simulink model "Intergration_ACC"  (R2018b)
settings: Solver=FixedStepDiscrete  StartTime=0.0  StopTime=inf  FixedStep=0.005  RelTol=1e-3
PostLoadFcn:
  | if any(exist('dsrtsu_mdlpostloadfcn', 'file') ~= 0), dsrtsu_mdlpostloadfcn('Execute', bdroot); end
values from neighbouring files (symbols this model uses):
  P_x165_On = 1.0    [CAN_Tx.sldd]
  P_x242_On = 1.0    [CAN_Tx.sldd]
  P_x246_On = 1.0    [CAN_Tx.sldd]
libraries: rtican x112, simulink x59
(part 25 of 31)

== system Intergration_ACC/TX/ESC_FrontWheelSpeedKPH_0x123 ==
  <WhlGndVelLDrvn_Radar> : Inport
  <WhlGndVelRDrvn_Radar> : Inport  Port=2
  <LDrvnWhlRotlDircn> : Inport  Port=3
  <RDrvnWhlRotlDircn> : Inport  Port=4
  Cast To Double{1..6} (6 alike) : DataTypeConversion  OutDataTypeStr=double
  Constant : Constant  Value=0  OutDataTypeStr=uint8
  Constant1 : Constant  Value=0  OutDataTypeStr=double
  Constant6 : Constant  Value=7  OutDataTypeStr=uint8
  ESC_FrontWheelSpeedKPH : rtican/RTICAN Transmit (TX)   Reserved1=[]  Reserved2=[]  Reserved3=[]  Reserved4=[]  SfcnMessage=[]  Msg_Struct=[]  BoardTypeNo=[]  BoardNo=[]  ChannelNo=[]  Parameters=[]  DialogFcn=[]  UnitName=[]  Revision=[]  UnitValues=[]  DSProperties=struct('RTI',struct('Version',uint32(5),'BlockType',struct('isSLSource',uint8(1),'isSLSink',uint8(1),'isHWSource',uint8(0),'isHWSink',uint8(0),'isSetup',uint8(0),'isInline',uint8(1),'isNonInline',uint8(0),'isInterrupt',uint8(0),'isChannelwise',uint8(0)),'IOBoardType','RTICAN','UnitType','MESSAGE','Identifier','TX','DialogType','MSVC','BlockSet','RTICAN','SlaveProcessor','CAN'))  RTIBlockInterface=struct('InputPortsWidth',int32([1 1 1 1 1 1 1 1 1 1]),'InputPortsActive',[1 1 1 1 1 1 1 1 1 1],'InputPortsName',{{'ESC_FrontWheelSpeedsKPH_Checksum','ESC_FrontWheelSpeedsKPH_AliveCou','ESC_Mcylinder_PressureInvalid','ESC_Mcylinder_Pressure','ESC_FRWheelSpeedInvalid','ESC_FRWheelDirection','ESC_FRWheelSpeedKPH','ESC_FLWheelSpeedInvalid','ESC_FLWheelDirection','ESC_FLWheelSpeedKPH'}},'InputPortsDataType',{{'SS_DOUBLE','SS_DOUBLE','SS_DOUBLE','SS_DOUBLE','SS_DOUBLE','SS_DOUBLE','SS_DOUBLE','SS_DOUBLE','SS_DOUBLE','SS_DOUBLE'}},'OutputPortsWidth',int32([1 1 1 1]),'OutputPortsActive',[1 1 1 1],'OutputPortsName',{{['TX status'],['TX time'],['TX delta time'],['TX delay time']}},'DialogFcn','rtican_message_interface_gui','BlockDisplay',{{'','center'}},'IconTransparency','on','InitLevel',3,'BlockName',struct('Token',{{'ESC_FrontWheelSpeedKPH'}}),'SampleTime',{{-1}},'TriggerPort',{{'none'}},'EnablePort',{{'none'}})  RTIBlockParameters=struct('BoardTypeNo',{{1,'OFF',[]}},'BoardNo',{{3,'ON',[1 16]}},'ChannelNo',{{2,'ON',[1 2]}},'Parameters',{{struct('DataFileSupport',struct('DataFileSelectedMaster',1,'DataFileSelectedLocal',1,'DataFileName','c:\users\administrator.zx-201607042142\documents\matlab\zone\dbc\ars410od_privatecan.dbc|c:\users\administrator.zx-201607042142\desktop\zone\2020_demo\410\asr410od_public_can.dbc|','DataFileDate',{{{''},{['30-十一月-2020 09:38:41']}}},'SelectedFile','..\..\..\..\..\desktop\zone\2020_demo\410\asr410od_public_can.dbc','InterfaceFcn','rtican_dbc_file_parser'),'Options',struct('StatusSelected',1,'TimeSelected',1,'DeltaTimeSelected',1,'DelayTimeSelected',1,'DelayTimeTXCommandSelected',0,'EncodeSetUnusedBitsToOne',0,'EnableMsgLoopback',0,'TriggerPort',struct('Selected',0,'TriggerType',0),'EnablePortSelected',0,'SignalOnPortnameSelected',1,'UserCoding',struct('Selected',0,'InterfaceFile','UserEncodingFile','FcnName','UserEncodeFcn','InportSelected',0,'InportWidth',1,'OutportSelected',0,'OutportWidth',1),'TerminationMsg',struct('Selected',0,'Byte0_7','0'),'InitialMsg',struct('Selected',0,'Byte0_7','0')),'Message',struct('MsgOnBlocknameSelected',1,'MsgName','ESC_FrontWheelSpeedKPH','MsgIdFormat',0,'MsgId',291,'MsgLength',8,'NumSignals',10,'SampleTime',-1,'StartTime',struct('Selected',0,'Value',3),'AutoRepeatTime',struct('Selected',0,'Value',0.1),'Timeout',struct('Selected',0,'Value',0.1),'DelayTime',struct('Selected',0,'Value',0.1),'Signal',struct('SgnName',{'ESC_FrontWheelSpeedsKPH_Checksum','ESC_FrontWheelSpeedsKPH_AliveCou','ESC_Mcylinder_PressureInvalid','ESC_Mcylinder_Pressure','ESC_FRWheelSpeedInvalid','ESC_FRWheelDirection','ESC_FRWheelSpeedKPH','ESC_FLWheelSpeedInvalid','ESC_FLWheelDirection','ESC_FLWheelSpeedKPH'},'SgnStartBit',{0,8,12,24,32,33,35,48,49,51},'SgnLength',{8,4,1,8,1,2,13,1,2,13},'SgnType',{0,0,0,0,0,0,0,0,0,0},'ModeValue',{-1,-1,-1,-1,-1,-1,-1,-1,-1,-1},'DataType',{0,0,0,0,0,0,0,0,0,0},'ByteLayout',{2,2,2,2,2,2,2,2,2,2},'Factor',{1,1,1,1,1,1,0.05625,1,1,0.05625},'Offset',{0,0,0,0,0,0,0,0,0,0},'SgnComment',{{'ESC_FrontWheelSpeedsKPH_Checksum'},{'ESC_FrontWheelSpeedsKPH_AliveCou'},{'ESC_Mcylinder_PressureInvalid'},{'ESC_Mcylinder_Pressure'},{'ESC_FRWheelSpeedInvalid'},{'ESC_FRWheelDirection'},{'ESC_FRWheelSpeedKPH'},{'ESC_FLWheelSpeedInvalid'},{'ESC_FLWheelDirection'},{'ESC_FLWheelSpeedKPH'}},'SgnUnit',{'','','','','','','','','',''},'Min',{0,0,0,0,0,0,0,0,0,0},'Max',{255,15,1,254,1,3,460.6875,1,3,460.6875},'SLDataType',{'SS_DOUBLE','SS_DOUBLE','SS_DOUBLE','SS_DOUBLE','SS_DOUBLE','SS_DOUBLE','SS_DOUBLE','SS_DOUBLE','SS_DOUBLE','SS_DOUBLE'}),'MsgIdNumFormat',1,'MsgComment',{{''}}),'Version',1.2,'general',struct('isFromLib',0)),'OFF',[]}},'GroupId',{{struct('Group',{{'RTICAN'}},'No',3,'Behavior',{{'NAMECHANGE'}},'BlockType',{{'SINK'}},'NameChangeFlag',0),'OFF',[]}},'SFcnRTICANMessage',{{struct('MsgType','TX','SFcnPortType','Scalar','MsgName','ESC_FrontWheelSpeedKPH','MsgIdFormat','STD','MsgId',291,'MsgLength',8,'NumSignals',10,'SampleTime',-1,'StartTime',struct('Selected','no','Value',3),'AutoRepeatTime',struct('Selected','no','Value',0.1),'Timeout',struct('Selected','no','Value',0.1),'Signal',struct('SgnName',{'ESC_FrontWheelSpeedsKPH_Checksum','ESC_FrontWheelSpeedsKPH_AliveCou','ESC_Mcylinder_PressureInvalid','ESC_Mcylinder_Pressure','ESC_FRWheelSpeedInvalid','ESC_FRWheelDirection','ESC_FRWheelSpeedKPH','ESC_FLWheelSpeedInvalid','ESC_FLWheelDirection','ESC_FLWheelSpeedKPH'},'SgnStartBit',{0,8,12,24,32,33,35,48,49,51},'SgnLength',{8,4,1,8,1,2,13,1,2,13},'SgnType',{'standard','standard','standard','standard','standard','standard','standard','standard','standard','standard'},'ModeValue',{-1,-1,-1,-1,-1,-1,-1,-1,-1,-1},'DataType',{['unsigned int'],['unsigned int'],['unsigned int'],['unsigned int'],['unsigned int'],['unsigned int'],['unsigned int'],['unsigned int'],['unsigned int'],['unsigned int']},'ByteLayout',{['motorola back.'],['motorola back.'],['motorola back.'],['motorola back.'],['motorola back.'],['motorola back.'],['motorola back.'],['motorola back.'],['motorola back.'],['motorola back.']},'Factor',{1,1,1,1,1,1,0.05625,1,1,0.05625},'Offset',{0,0,0,0,0,0,0,0,0,0},'SLDataType',{'SS_DOUBLE','SS_DOUBLE','SS_DOUBLE','SS_DOUBLE','SS_DOUBLE','SS_DOUBLE','SS_DOUBLE','SS_DOUBLE','SS_DOUBLE','SS_DOUBLE'}),'StatusSelected','yes','TimeSelected','yes','DeltaTimeSelected','yes','DelayTimeSelected','yes','DelayTimeTXCommandSelected','no','EncodeSetUnusedBitsToOne','no','EnableMsgLoopback','no','TriggerPort',struct('Selected','no','TriggerType',0),'EnablePortSelected','no','UserCoding',struct('Selected','no','InterfaceFile','UserEncodingFile','FcnName','UserEncodeFcn','InportSelected','no','InportWidth',1,'OutportSelected','no','OutportWidth',1),'TerminationMsg',struct('Selected','no','Byte0','0x00','Byte1','0x00','Byte2','0x00','Byte3','0x00','Byte4','0x00','Byte5','0x00','Byte6','0x00','Byte7','0x00'),'InitialMsg',struct('Selected','no','Byte0','0x00','Byte1','0x00','Byte2','0x00','Byte3','0x00','Byte4','0x00','Byte5','0x00','Byte6','0x00','Byte7','0x00'),'BoardType','DS1','BoardNo',3,'ControllerNo',2),'OFF',[]}},'TLCFileName',{{'rtican_tx_message','OFF',[]}})  RTISFcnParameters=struct('SFcnRTICANMessage','struct','TLCFileName','char')  RTIBlockParaDefault=struct('BoardTypeNo',4302,'BoardNo',1,'ChannelNo',1,'Parameters',struct('DataFileSupport',struct('DataFileSelectedMaster',0,'DataFileSelectedLocal',0,'DataFileName','','DataFileDate','','SelectedFile',['<no file selected>']),'Options',struct('StatusSelected',1,'TimeSelected',1,'DeltaTimeSelected',1,'DelayTimeSelected',1,'DelayTimeTXCommandSelected',0,'EncodeSetUnusedBitsToOne',0,'EnableMsgLoopback',0,'TriggerPort',struct('Selected',0,'TriggerType','rising'),'EnablePortSelected',0,'SignalOnPortnameSelected',1,'UserCoding',struct('Selected',0,'InterfaceFile','UserEncodingFile','FcnName','UserEncodeFcn','InportSelected',0,'InportWidth',1,'OutportSelected',0,'OutportWidth',1),'TerminationMsg',struct('Selected',0,'Byte0_7','0'),'InitialMsg',struct('Selected',0,'Byte0_7','0')),'Message',struct('MsgOnBlocknameSelected',0,'MsgName',['TX Message'],'MsgIdFormat',0,'MsgId',100,'MsgLength',8,'NumSignals',1,'SampleTime',-1,'StartTime',struct('Selected',0,'Value',0),'AutoRepeatTime',struct('Selected',0,'Value',0.1),'Timeout',struct('Selected',0,'Value',0.1),'DelayTime',struct('Selected',0,'Value',0.1),'Signal',struct('SgnName',['TX signal'],'SgnStartBit',0,'SgnLength',8,'SgnType',0,'ModeValue',-1,'DataType',0,'SLDataType','SS_DOUBLE','ByteLayout',0,'Factor',1,'Offset',0,'Min',0,'Max',255,'SgnComment',{{}},'SgnUnit',''),'MsgIdNumFormat',0,'MsgComment',{{''}}),'Version',1.2,'general',struct('isFromLib',1)),'GroupId',struct('Group',{{'RTICAN'}},'No',1,'Behavior',{{'NAMECHANGE'}},'BlockType',{{'SINK'}},'NameChangeFlag',0),'SFcnRTICANMessage',struct('MsgType','TX','MsgName',['TX Message'],'MsgIdFormat','STD','MsgId',100,'MsgLength',2,'NumSignals',1,'SampleTime',-1,'StartTime',struct('Selected','no','Value',0),'AutoRepeatTime',struct('Selected','no','Value',0.1),'Timeout',struct('Selected','no','Value',0.1),'DelayTime',struct('Selected','no','Value',0.1),'Signal',struct('SgnName',['TX signal'],'SgnStartBit',0,'SgnLength',8,'SgnType','standard','ModeValue',-1,'DataType',['unsigned int'],'ByteLayout',['little endian'],'SLDataType','SS_DOUBLE','Factor',1,'Offset',0),'StatusSelected','yes','TimeSelected','yes','DeltaTimeSelected','yes','DelayTimeSelected','yes','EnablePortSelected','no','EnableMsgLoopback','no','DelayTimeTXCommandSelected','no','EncodeSetUnusedBitsToOne','no','UserCoding',struct('Selected','no','InterfaceFile','UserDecodingFile','FcnName','UserDecodeFcn','InportSelected','no','InportWidth',1,'OutportSelected','no','OutportWidth',1),'TerminationMsg',struct('Selected','no','Byte0','0x00','Byte1','0x00','Byte2','0x00','Byte3','0x00','Byte4','0x00','Byte5','0x00','Byte6','0x00','Byte7','0x00'),'InitialMsg',struct('Selected','no','Byte0','0x00','Byte1','0x00','Byte2','0x00','Byte3','0x00','Byte4','0x00','Byte5','0x00','Byte6','0x00','Byte7','0x00'),'TriggerPort',struct('Selected','no','TriggerType','rising'),'BoardType','DS4302','BoardNo',1,'ControllerNo',1,'SFcnPortType','Scalar'),'TLCFileName','rtican_tx_message')
      settings: AttributesFormatString=Group Id: RTICAN3\n  SourceProductName=dSPACE RTI CAN Blockset
  RollingCounter1 : Subsystem
  S-Function Builder1 : S-Function  InitFcn=try, set_param(gcb,'FunctionName','CheckSum_Tx_Radar410'), end  FunctionName=CheckSum_Tx_Radar410  SFunctionModules=CheckSum_Tx_Radar410_wrapper  SFunctionDeploymentMode=off  EnableBusSupport=off  mask(S-Function Builder){}
      mask help: Simulink:masks:SFunctionBuilder_MD
      mask init: same as Intergration_ACC/Tx_410_10ms/S-Function Builder1
      settings: CopyFcn=set_param(gcbh,'LinkStatus','none')  PreSaveFcn=try, set_param(gcb,'FunctionName','CheckSum_Tx_Radar410'), end  OpenFcn=sfunctionwizard(gcbh)
      mask Display: plot(val(:,1),val(:,2)),disp(sys), port_label('input',1,'data'), port_label('input',2,'length'), port_label('output',1,'u8_crc8')
  Subsystem : Subsystem
  Subsystem1 : Subsystem
  Subsystem2 : Subsystem
  Subsystem3 : Subsystem
  Subsystem4 : Subsystem
  Vector Concatenate1 : Concatenate  NumInputs=7
  wires:
  Subsystem2/1(Out1) -> Cast To Double1/1
  <LDrvnWhlRotlDircn>/1 -> Cast To Double2/1, Subsystem1/2(<LDrvnWhlRotlDircn>)
  Subsystem4/1(Byte6) -> Vector Concatenate1/7
  Cast To Double1/1 -> ESC_FrontWheelSpeedKPH/7
  Constant1/1 -> ESC_FrontWheelSpeedKPH/3, ESC_FrontWheelSpeedKPH/8, ESC_FrontWheelSpeedKPH/5, ESC_FrontWheelSpeedKPH/4
  Vector Concatenate1/1 -> S-Function Builder1/1
  <WhlGndVelRDrvn_Radar>/1 -> Subsystem2/1(<WhlGndVelLDrvn_Radar>)
  <RDrvnWhlRotlDircn>/1 -> Cast To Double4/1, Subsystem3/2(<LDrvnWhlRotlDircn>)
  Cast To Double6/1 -> ESC_FrontWheelSpeedKPH/1
  Subsystem/3(Output) -> Subsystem1/1(In1)
  Subsystem2/3(Output) -> Subsystem3/1(In1)
  Subsystem2/2(Byte2) -> Vector Concatenate1/3
  RollingCounter1/1(RC) -> Cast To Double5/1, Subsystem4/1(In1)
  <WhlGndVelLDrvn_Radar>/1 -> Subsystem/1(<WhlGndVelLDrvn_Radar>)
  Subsystem1/1(Byte1) -> Vector Concatenate1/2
  Constant/1 -> Vector Concatenate1/6, Vector Concatenate1/5
  Cast To Double3/1 -> ESC_FrontWheelSpeedKPH/10
  Constant6/1 -> S-Function Builder1/2
  Cast To Double4/1 -> ESC_FrontWheelSpeedKPH/6
  Cast To Double2/1 -> ESC_FrontWheelSpeedKPH/9
  S-Function Builder1/1 -> Cast To Double6/1
  Subsystem/2(Byte0) -> Vector Concatenate1/1
  Subsystem3/1(Byte3) -> Vector Concatenate1/4
  Cast To Double5/1 -> ESC_FrontWheelSpeedKPH/2
  Subsystem/1(Out1) -> Cast To Double3/1

== system Intergration_ACC/TX/ESC_RearWheelSpeedKPH_0x124 ==
  <WhlGndVelLNonDrvn_Radar> : Inport
  <WhlGndVelRNonDrvn_Radar> : Inport  Port=2
  <LNonDrvnWhlRotlDircn_Radar> : Inport  Port=3
  <RNonDrvnWhlRotlDircn_Radar> : Inport  Port=4
  Cast To Double{1..6} (6 alike) : DataTypeConversion  OutDataTypeStr=double
  Constant : Constant  Value=0  OutDataTypeStr=uint8
  Constant1 : Constant  Value=0  OutDataTypeStr=double
  Constant6 : Constant  Value=7  OutDataTypeStr=uint8
  ESC_RearWheelSpeedKPH : rtican/RTICAN Transmit (TX)   Reserved1=[]  Reserved2=[]  Reserved3=[]  Reserved4=[]  SfcnMessage=[]  Msg_Struct=[]  BoardTypeNo=[]  BoardNo=[]  ChannelNo=[]  Parameters=[]  DialogFcn=[]  UnitName=[]  Revision=[]  UnitValues=[]  DSProperties=struct('RTI',struct('Version',uint32(5),'BlockType',struct('isSLSource',uint8(1),'isSLSink',uint8(1),'isHWSource',uint8(0),'isHWSink',uint8(0),'isSetup',uint8(0),'isInline',uint8(1),'isNonInline',uint8(0),'isInterrupt',uint8(0),'isChannelwise',uint8(0)),'IOBoardType','RTICAN','UnitType','MESSAGE','Identifier','TX','DialogType','MSVC','BlockSet','RTICAN','SlaveProcessor','CAN'))  RTIBlockInterface=struct('InputPortsWidth',int32([1 1 1 1 1 1 1 1]),'InputPortsActive',[1 1 1 1 1 1 1 1],'InputPortsName',{{'ESC_RearWheelSpeedsKPH_Checksum','ESC_RearWheelSpeedsKPH_AliveCoun','ESC_RRWheelSpeedInvalid','ESC_RRWheelDirection','ESC_RRWheelSpeedKPH','ESC_RLWheelSpeedInvalid','ESC_RLWheelDirection','ESC_RLWheelSpeedKPH'}},'InputPortsDataType',{{'SS_DOUBLE','SS_DOUBLE','SS_DOUBLE','SS_DOUBLE','SS_DOUBLE','SS_DOUBLE','SS_DOUBLE','SS_DOUBLE'}},'OutputPortsWidth',int32([1 1 1 1]),'OutputPortsActive',[1 1 1 1],'OutputPortsName',{{['TX status'],['TX time'],['TX delta time'],['TX delay time']}},'DialogFcn','rtican_message_interface_gui','BlockDisplay',{{'','center'}},'IconTransparency','on','InitLevel',3,'BlockName',struct('Token',{{'ESC_RearWheelSpeedKPH'}}),'SampleTime',{{-1}},'TriggerPort',{{'none'}},'EnablePort',{{'none'}})  RTIBlockParameters=struct('BoardTypeNo',{{1,'OFF',[]}},'BoardNo',{{3,'ON',[1 16]}},'ChannelNo',{{2,'ON',[1 2]}},'Parameters',{{struct('DataFileSupport',struct('DataFileSelectedMaster',1,'DataFileSelectedLocal',1,'DataFileName','c:\users\administrator.zx-201607042142\documents\matlab\zone\dbc\ars410od_privatecan.dbc|c:\users\administrator.zx-201607042142\desktop\zone\2020_demo\410\asr410od_public_can.dbc|','DataFileDate',{{{''},{['30-十一月-2020 09:38:41']}}},'SelectedFile','..\..\..\..\..\desktop\zone\2020_demo\410\asr410od_public_can.dbc','InterfaceFcn','rtican_dbc_file_parser'),'Options',struct('StatusSelected',1,'TimeSelected',1,'DeltaTimeSelected',1,'DelayTimeSelected',1,'DelayTimeTXCommandSelected',0,'EncodeSetUnusedBitsToOne',0,'EnableMsgLoopback',0,'TriggerPort',struct('Selected',0,'TriggerType',0),'EnablePortSelected',0,'SignalOnPortnameSelected',1,'UserCoding',struct('Selected',0,'InterfaceFile','UserEncodingFile','FcnName','UserEncodeFcn','InportSelected',0,'InportWidth',1,'OutportSelected',0,'OutportWidth',1),'TerminationMsg',struct('Selected',0,'Byte0_7','0'),'InitialMsg',struct('Selected',0,'Byte0_7','0')),'Message',struct('MsgOnBlocknameSelected',1,'MsgName','ESC_RearWheelSpeedKPH','MsgIdFormat',0,'MsgId',292,'MsgLength',8,'NumSignals',8,'SampleTime',-1,'StartTime',struct('Selected',0,'Value',3),'AutoRepeatTime',struct('Selected',0,'Value',0.1),'Timeout',struct('Selected',0,'Value',0.1),'DelayTime',struct('Selected',0,'Value',0.1),'Signal',struct('SgnName',{'ESC_RearWheelSpeedsKPH_Checksum','ESC_RearWheelSpeedsKPH_AliveCoun','ESC_RRWheelSpeedInvalid','ESC_RRWheelDirection','ESC_RRWheelSpeedKPH','ESC_RLWheelSpeedInvalid','ESC_RLWheelDirection','ESC_RLWheelSpeedKPH'},'SgnStartBit',{0,8,32,33,35,48,49,51},'SgnLength',{8,4,1,2,13,1,2,13},'SgnType',{0,0,0,0,0,0,0,0},'ModeValue',{-1,-1,-1,-1,-1,-1,-1,-1},'DataType',{0,0,0,0,0,0,0,0},'ByteLayout',{2,2,2,2,2,2,2,2},'Factor',{1,1,1,1,0.05625,1,1,0.05625},'Offset',{0,0,0,0,0,0,0,0},'SgnComment',{{'ESC_RearWheelSpeedsKPH_Checksum'},{'ESC_RearWheelSpeedsKPH_AliveCoun'},{'ESC_RRWheelSpeedInvalid'},{'ESC_RRWheelDirection'},{'ESC_RRWheelSpeedKPH'},{'ESC_RLWheelSpeedInvalid'},{'ESC_RLWheelDirection'},{'ESC_RLWheelSpeedKPH'}},'SgnUnit',{'','','','','','','',''},'Min',{0,0,0,0,0,0,0,0},'Max',{255,15,1,3,460.6875,1,1,460.6875},'SLDataType',{'SS_DOUBLE','SS_DOUBLE','SS_DOUBLE','SS_DOUBLE','SS_DOUBLE','SS_DOUBLE','SS_DOUBLE','SS_DOUBLE'}),'MsgIdNumFormat',1,'MsgComment',{{''}}),'Version',1.2,'general',struct('isFromLib',0)),'OFF',[]}},'GroupId',{{struct('Group',{{'RTICAN'}},'No',3,'Behavior',{{'NAMECHANGE'}},'BlockType',{{'SINK'}},'NameChangeFlag',0),'OFF',[]}},'SFcnRTICANMessage',{{struct('MsgType','TX','SFcnPortType','Scalar','MsgName','ESC_RearWheelSpeedKPH','MsgIdFormat','STD','MsgId',292,'MsgLength',8,'NumSignals',8,'SampleTime',-1,'StartTime',struct('Selected','no','Value',3),'AutoRepeatTime',struct('Selected','no','Value',0.1),'Timeout',struct('Selected','no','Value',0.1),'Signal',struct('SgnName',{'ESC_RearWheelSpeedsKPH_Checksum','ESC_RearWheelSpeedsKPH_AliveCoun','ESC_RRWheelSpeedInvalid','ESC_RRWheelDirection','ESC_RRWheelSpeedKPH','ESC_RLWheelSpeedInvalid','ESC_RLWheelDirection','ESC_RLWheelSpeedKPH'},'SgnStartBit',{0,8,32,33,35,48,49,51},'SgnLength',{8,4,1,2,13,1,2,13},'SgnType',{'standard','standard','standard','standard','standard','standard','standard','standard'},'ModeValue',{-1,-1,-1,-1,-1,-1,-1,-1},'DataType',{['unsigned int'],['unsigned int'],['unsigned int'],['unsigned int'],['unsigned int'],['unsigned int'],['unsigned int'],['unsigned int']},'ByteLayout',{['motorola back.'],['motorola back.'],['motorola back.'],['motorola back.'],['motorola back.'],['motorola back.'],['motorola back.'],['motorola back.']},'Factor',{1,1,1,1,0.05625,1,1,0.05625},'Offset',{0,0,0,0,0,0,0,0},'SLDataType',{'SS_DOUBLE','SS_DOUBLE','SS_DOUBLE','SS_DOUBLE','SS_DOUBLE','SS_DOUBLE','SS_DOUBLE','SS_DOUBLE'}),'StatusSelected','yes','TimeSelected','yes','DeltaTimeSelected','yes','DelayTimeSelected','yes','DelayTimeTXCommandSelected','no','EncodeSetUnusedBitsToOne','no','EnableMsgLoopback','no','TriggerPort',struct('Selected','no','TriggerType',0),'EnablePortSelected','no','UserCoding',struct('Selected','no','InterfaceFile','UserEncodingFile','FcnName','UserEncodeFcn','InportSelected','no','InportWidth',1,'OutportSelected','no','OutportWidth',1),'TerminationMsg',struct('Selected','no','Byte0','0x00','Byte1','0x00','Byte2','0x00','Byte3','0x00','Byte4','0x00','Byte5','0x00','Byte6','0x00','Byte7','0x00'),'InitialMsg',struct('Selected','no','Byte0','0x00','Byte1','0x00','Byte2','0x00','Byte3','0x00','Byte4','0x00','Byte5','0x00','Byte6','0x00','Byte7','0x00'),'BoardType','DS1','BoardNo',3,'ControllerNo',2),'OFF',[]}},'TLCFileName',{{'rtican_tx_message','OFF',[]}})  RTISFcnParameters=struct('SFcnRTICANMessage','struct','TLCFileName','char')  RTIBlockParaDefault=struct('BoardTypeNo',4302,'BoardNo',1,'ChannelNo',1,'Parameters',struct('DataFileSupport',struct('DataFileSelectedMaster',0,'DataFileSelectedLocal',0,'DataFileName','','DataFileDate','','SelectedFile',['<no file selected>']),'Options',struct('StatusSelected',1,'TimeSelected',1,'DeltaTimeSelected',1,'DelayTimeSelected',1,'DelayTimeTXCommandSelected',0,'EncodeSetUnusedBitsToOne',0,'EnableMsgLoopback',0,'TriggerPort',struct('Selected',0,'TriggerType','rising'),'EnablePortSelected',0,'SignalOnPortnameSelected',1,'UserCoding',struct('Selected',0,'InterfaceFile','UserEncodingFile','FcnName','UserEncodeFcn','InportSelected',0,'InportWidth',1,'OutportSelected',0,'OutportWidth',1),'TerminationMsg',struct('Selected',0,'Byte0_7','0'),'InitialMsg',struct('Selected',0,'Byte0_7','0')),'Message',struct('MsgOnBlocknameSelected',0,'MsgName',['TX Message'],'MsgIdFormat',0,'MsgId',100,'MsgLength',8,'NumSignals',1,'SampleTime',-1,'StartTime',struct('Selected',0,'Value',0),'AutoRepeatTime',struct('Selected',0,'Value',0.1),'Timeout',struct('Selected',0,'Value',0.1),'DelayTime',struct('Selected',0,'Value',0.1),'Signal',struct('SgnName',['TX signal'],'SgnStartBit',0,'SgnLength',8,'SgnType',0,'ModeValue',-1,'DataType',0,'SLDataType','SS_DOUBLE','ByteLayout',0,'Factor',1,'Offset',0,'Min',0,'Max',255,'SgnComment',{{}},'SgnUnit',''),'MsgIdNumFormat',0,'MsgComment',{{''}}),'Version',1.2,'general',struct('isFromLib',1)),'GroupId',struct('Group',{{'RTICAN'}},'No',1,'Behavior',{{'NAMECHANGE'}},'BlockType',{{'SINK'}},'NameChangeFlag',0),'SFcnRTICANMessage',struct('MsgType','TX','MsgName',['TX Message'],'MsgIdFormat','STD','MsgId',100,'MsgLength',2,'NumSignals',1,'SampleTime',-1,'StartTime',struct('Selected','no','Value',0),'AutoRepeatTime',struct('Selected','no','Value',0.1),'Timeout',struct('Selected','no','Value',0.1),'DelayTime',struct('Selected','no','Value',0.1),'Signal',struct('SgnName',['TX signal'],'SgnStartBit',0,'SgnLength',8,'SgnType','standard','ModeValue',-1,'DataType',['unsigned int'],'ByteLayout',['little endian'],'SLDataType','SS_DOUBLE','Factor',1,'Offset',0),'StatusSelected','yes','TimeSelected','yes','DeltaTimeSelected','yes','DelayTimeSelected','yes','EnablePortSelected','no','EnableMsgLoopback','no','DelayTimeTXCommandSelected','no','EncodeSetUnusedBitsToOne','no','UserCoding',struct('Selected','no','InterfaceFile','UserDecodingFile','FcnName','UserDecodeFcn','InportSelected','no','InportWidth',1,'OutportSelected','no','OutportWidth',1),'TerminationMsg',struct('Selected','no','Byte0','0x00','Byte1','0x00','Byte2','0x00','Byte3','0x00','Byte4','0x00','Byte5','0x00','Byte6','0x00','Byte7','0x00'),'InitialMsg',struct('Selected','no','Byte0','0x00','Byte1','0x00','Byte2','0x00','Byte3','0x00','Byte4','0x00','Byte5','0x00','Byte6','0x00','Byte7','0x00'),'TriggerPort',struct('Selected','no','TriggerType','rising'),'BoardType','DS4302','BoardNo',1,'ControllerNo',1,'SFcnPortType','Scalar'),'TLCFileName','rtican_tx_message')
      settings: AttributesFormatString=Group Id: RTICAN3\n  SourceProductName=dSPACE RTI CAN Blockset
  RollingCounter1 : Subsystem
  S-Function Builder1 : S-Function  InitFcn=try, set_param(gcb,'FunctionName','CheckSum_Tx_Radar410'), end  FunctionName=CheckSum_Tx_Radar410  SFunctionModules=CheckSum_Tx_Radar410_wrapper  SFunctionDeploymentMode=off  EnableBusSupport=off  mask(S-Function Builder){}
      mask help: Simulink:masks:SFunctionBuilder_MD
      mask init: same as Intergration_ACC/Tx_410_10ms/S-Function Builder1
      settings: CopyFcn=set_param(gcbh,'LinkStatus','none')  PreSaveFcn=try, set_param(gcb,'FunctionName','CheckSum_Tx_Radar410'), end  OpenFcn=sfunctionwizard(gcbh)
      mask Display: plot(val(:,1),val(:,2)),disp(sys), port_label('input',1,'data'), port_label('input',2,'length'), port_label('output',1,'u8_crc8')
  Subsystem : Subsystem
  Subsystem1 : Subsystem
  Subsystem2 : Subsystem
  Subsystem3 : Subsystem
  Subsystem4 : Subsystem
  Vector Concatenate1 : Concatenate  NumInputs=7
  wires:
  Cast To Double3/1 -> ESC_RearWheelSpeedKPH/4
  Subsystem/1(Out1) -> Cast To Double4/1
  Subsystem2/3(Output) -> Subsystem3/1(In1)
  <LNonDrvnWhlRotlDircn_Radar>/1 -> Subsystem1/2(<LDrvnWhlRotlDircn>), Cast To Double2/1
  <WhlGndVelLNonDrvn_Radar>/1 -> Subsystem/1(<WhlGndVelLDrvn_Radar>)
  <RNonDrvnWhlRotlDircn_Radar>/1 -> Cast To Double3/1, Subsystem3/2(<LDrvnWhlRotlDircn>)
  Subsystem2/1(Out1) -> Cast To Double1/1
  Subsystem/3(Output) -> Subsystem1/1(In1)
  Cast To Double6/1 -> ESC_RearWheelSpeedKPH/1
  <WhlGndVelRNonDrvn_Radar>/1 -> Subsystem2/1(<WhlGndVelLDrvn_Radar>)
  Constant1/1 -> ESC_RearWheelSpeedKPH/6, ESC_RearWheelSpeedKPH/3
  Subsystem4/1(Byte6) -> Vector Concatenate1/7
  Cast To Double5/1 -> ESC_RearWheelSpeedKPH/2
  Cast To Double4/1 -> ESC_RearWheelSpeedKPH/8
  S-Function Builder1/1 -> Cast To Double6/1
  Constant6/1 -> S-Function Builder1/2
  RollingCounter1/1(RC) -> Cast To Double5/1, Subsystem4/1(In1)
  Subsystem2/2(Byte2) -> Vector Concatenate1/3
  Vector Concatenate1/1 -> S-Function Builder1/1
  Constant/1 -> Vector Concatenate1/6, Vector Concatenate1/5
  Subsystem3/1(Byte3) -> Vector Concatenate1/4
  Subsystem/2(Byte0) -> Vector Concatenate1/1
  Cast To Double2/1 -> ESC_RearWheelSpeedKPH/7
  Subsystem1/1(Byte1) -> Vector Concatenate1/2
  Cast To Double1/1 -> ESC_RearWheelSpeedKPH/5

== system Intergration_ACC/TX/ESC_Status_0x126 ==
  <VehSpdAvg> : Inport
  Cast To Double1 : DataTypeConversion  OutDataTypeStr=double
  Cast To Double2 : DataTypeConversion  OutDataTypeStr=double
  Cast To Double4 : DataTypeConversion  OutDataTypeStr=double
  Constant : Constant  Value=0  OutDataTypeStr=uint8
  Constant1 : Constant  Value=0  OutDataTypeStr=double
  Constant6 : Constant  Value=7  OutDataTypeStr=uint8
  ESC_Status : rtican/RTICAN Transmit (TX)   Reserved1=[]  Reserved2=[]  Reserved3=[]  Reserved4=[]  SfcnMessage=[]  Msg_Struct=[]  BoardTypeNo=[]  BoardNo=[]  ChannelNo=[]  Parameters=[]  DialogFcn=[]  UnitName=[]  Revision=[]  UnitValues=[]  DSProperties=struct('RTI',struct('Version',uint32(5),'BlockType',struct('isSLSource',uint8(1),'isSLSink',uint8(1),'isHWSource',uint8(0),'isHWSink',uint8(0),'isSetup',uint8(0),'isInline',uint8(1),'isNonInline',uint8(0),'isInterrupt',uint8(0),'isChannelwise',uint8(0)),'IOBoardType','RTICAN','UnitType','MESSAGE','Identifier','TX','DialogType','MSVC','BlockSet','RTICAN','SlaveProcessor','CAN'))  RTIBlockInterface=struct('InputPortsWidth',int32([1 1 1 1 1 1 1 1 1 1 1 1 1 1]),'InputPortsActive',ones(1,14),'InputPortsName',{{'ESC_Status_Checksum','ESC_Status_AliveCounter','ESC_HHCActive','ESC_AVHStatus','ESC_EPBStatus','ESC_BrakePedalSwitchInvalid','ESC_PATAResponse','ESC_VehicleSpeedInvalid','ESC_VehicleSpeed','ESC_ABSActive','ESC_BrakePedalSwitchStatus','ESC_TCSActive','ESC_ESPActive','ESC_ESPFailed'}},'InputPortsDataType',{{'SS_DOUBLE','SS_DOUBLE','SS_DOUBLE','SS_DOUBLE','SS_DOUBLE','SS_DOUBLE','SS_DOUBLE','SS_DOUBLE','SS_DOUBLE','SS_DOUBLE','SS_DOUBLE','SS_DOUBLE','SS_DOUBLE','SS_DOUBLE'}},'OutputPortsWidth',int32([1 1 1 1]),'OutputPortsActive',[1 1 1 1],'OutputPortsName',{{['TX status'],['TX time'],['TX delta time'],['TX delay time']}},'DialogFcn','rtican_message_interface_gui','BlockDisplay',{{'','center'}},'IconTransparency','on','InitLevel',3,'BlockName',struct('Token',{{'ESC_Status'}}),'SampleTime',{{-1}},'TriggerPort',{{'none'}},'EnablePort',{{'none'}})  RTIBlockParameters=struct('BoardTypeNo',{{1,'OFF',[]}},'BoardNo',{{3,'ON',[1 16]}},'ChannelNo',{{2,'ON',[1 2]}},'Parameters',{{struct('DataFileSupport',struct('DataFileSelectedMaster',1,'DataFileSelectedLocal',1,'DataFileName','c:\users\administrator.zx-201607042142\documents\matlab\zone\dbc\ars410od_privatecan.dbc|c:\users\administrator.zx-201607042142\desktop\zone\2020_demo\410\asr410od_public_can.dbc|','DataFileDate',{{{''},{['30-十一月-2020 09:38:41']}}},'SelectedFile','..\..\..\..\..\desktop\zone\2020_demo\410\asr410od_public_can.dbc','InterfaceFcn','rtican_dbc_file_parser'),'Options',struct('StatusSelected',1,'TimeSelected',1,'DeltaTimeSelected',1,'DelayTimeSelected',1,'DelayTimeTXCommandSelected',0,'EncodeSetUnusedBitsToOne',0,'EnableMsgLoopback',0,'TriggerPort',struct('Selected',0,'TriggerType',0),'EnablePortSelected',0,'SignalOnPortnameSelected',1,'UserCoding',struct('Selected',0,'InterfaceFile','UserEncodingFile','FcnName','UserEncodeFcn','InportSelected',0,'InportWidth',1,'OutportSelected',0,'OutportWidth',1),'TerminationMsg',struct('Selected',0,'Byte0_7','0'),'InitialMsg',struct('Selected',0,'Byte0_7','0')),'Message',struct('MsgOnBlocknameSelected',1,'MsgName','ESC_Status','MsgIdFormat',0,'MsgId',294,'MsgLength',8,'NumSignals',14,'SampleTime',-1,'StartTime',struct('Selected',0,'Value',3),'AutoRepeatTime',struct('Selected',0,'Value',0.1),'Timeout',struct('Selected',0,'Value',0.1),'DelayTime',struct('Selected',0,'Value',0.1),'Signal',struct('SgnName',{'ESC_Status_Checksum','ESC_Status_AliveCounter','ESC_HHCActive','ESC_AVHStatus','ESC_EPBStatus','ESC_BrakePedalSwitchInvalid','ESC_PATAResponse','ESC_VehicleSpeedInvalid','ESC_VehicleSpeed','ESC_ABSActive','ESC_BrakePedalSwitchStatus','ESC_TCSActive','ESC_ESPActive','ESC_ESPFailed'},'SgnStartBit',{0,8,16,33,35,38,40,42,43,56,57,60,61,63},'SgnLength',{8,4,1,2,2,1,1,1,13,1,1,1,1,1},'SgnType',{0,0,0,0,0,0,0,0,0,0,0,0,0,0},'ModeValue',{-1,-1,-1,-1,-1,-1,-1,-1,-1,-1,-1,-1,-1,-1},'DataType',{0,0,0,0,0,0,0,0,0,0,0,0,0,0},'ByteLayout',{2,2,2,2,2,2,2,2,2,2,2,2,2,2},'Factor',{1,1,1,1,1,1,1,1,0.05625,1,1,1,1,1},'Offset',{0,0,0,0,0,0,0,0,0,0,0,0,0,0},'SgnComment',{{'ESC_Status_Checksum'},{'ESC_Status_AliveCounter'},{'ESC_HHCActive'},{'ESC_AVHStatus'},{'ESC_EPBStatus'},{'ESC_BrakePedalSwitchInvalid'},{'ESC_PATAResponse'},{'ESC_VehicleSpeedInvalid'},{'ESC_VehicleSpeed'},{'ESC_ABSActive'},{'ESC_BrakePedalSwitchStatus'},{'ESC_TCSActive'},{'ESC_ESPActive'},{'ESC_ESPFailed'}},'SgnUnit',{'','','','','','','','','','','','','',''},'Min',{0,0,0,0,0,0,0,0,0,0,0,0,0,0},'Max',{255,15,1,3,3,1,1,1,460.6875,1,1,1,1,1},'SLDataType',{'SS_DOUBLE','SS_DOUBLE','SS_DOUBLE','SS_DOUBLE','SS_DOUBLE','SS_DOUBLE','SS_DOUBLE','SS_DOUBLE','SS_DOUBLE','SS_DOUBLE','SS_DOUBLE','SS_DOUBLE','SS_DOUBLE','SS_DOUBLE'}),'MsgIdNumFormat',1,'MsgComment',{{''}}),'Version',1.2,'general',struct('isFromLib',0)),'OFF',[]}},'GroupId',{{struct('Group',{{'RTICAN'}},'No',3,'Behavior',{{'NAMECHANGE'}},'BlockType',{{'SINK'}},'NameChangeFlag',0),'OFF',[]}},'SFcnRTICANMessage',{{struct('MsgType','TX','SFcnPortType','Scalar','MsgName','ESC_Status','MsgIdFormat','STD','MsgId',294,'MsgLength',8,'NumSignals',14,'SampleTime',-1,'StartTime',struct('Selected','no','Value',3),'AutoRepeatTime',struct('Selected','no','Value',0.1),'Timeout',struct('Selected','no','Value',0.1),'Signal',struct('SgnName',{'ESC_Status_Checksum','ESC_Status_AliveCounter','ESC_HHCActive','ESC_AVHStatus','ESC_EPBStatus','ESC_BrakePedalSwitchInvalid','ESC_PATAResponse','ESC_VehicleSpeedInvalid','ESC_VehicleSpeed','ESC_ABSActive','ESC_BrakePedalSwitchStatus','ESC_TCSActive','ESC_ESPActive','ESC_ESPFailed'},'SgnStartBit',{0,8,16,33,35,38,40,42,43,56,57,60,61,63},'SgnLength',{8,4,1,2,2,1,1,1,13,1,1,1,1,1},'SgnType',{'standard','standard','standard','standard','standard','standard','standard','standard','standard','standard','standard','standard','standard','standard'},'ModeValue',{-1,-1,-1,-1,-1,-1,-1,-1,-1,-1,-1,-1,-1,-1},'DataType',{['unsigned int'],['unsigned int'],['unsigned int'],['unsigned int'],['unsigned int'],['unsigned int'],['unsigned int'],['unsigned int'],['unsigned int'],['unsigned int'],['unsigned int'],['unsigned int'],['unsigned int'],['unsigned int']},'ByteLayout',{['motorola back.'],['motorola back.'],['motorola back.'],['motorola back.'],['motorola back.'],['motorola back.'],['motorola back.'],['motorola back.'],['motorola back.'],['motorola back.'],['motorola back.'],['motorola back.'],['motorola back.'],['motorola back.']},'Factor',{1,1,1,1,1,1,1,1,0.05625,1,1,1,1,1},'Offset',{0,0,0,0,0,0,0,0,0,0,0,0,0,0},'SLDataType',{'SS_DOUBLE','SS_DOUBLE','SS_DOUBLE','SS_DOUBLE','SS_DOUBLE','SS_DOUBLE','SS_DOUBLE','SS_DOUBLE','SS_DOUBLE','SS_DOUBLE','SS_DOUBLE','SS_DOUBLE','SS_DOUBLE','SS_DOUBLE'}),'StatusSelected','yes','TimeSelected','yes','DeltaTimeSelected','yes','DelayTimeSelected','yes','DelayTimeTXCommandSelected','no','EncodeSetUnusedBitsToOne','no','EnableMsgLoopback','no','TriggerPort',struct('Selected','no','TriggerType',0),'EnablePortSelected','no','UserCoding',struct('Selected','no','InterfaceFile','UserEncodingFile','FcnName','UserEncodeFcn','InportSelected','no','InportWidth',1,'OutportSelected','no','OutportWidth',1),'TerminationMsg',struct('Selected','no','Byte0','0x00','Byte1','0x00','Byte2','0x00','Byte3','0x00','Byte4','0x00','Byte5','0x00','Byte6','0x00','Byte7','0x00'),'InitialMsg',struct('Selected','no','Byte0','0x00','Byte1','0x00','Byte2','0x00','Byte3','0x00','Byte4','0x00','Byte5','0x00','Byte6','0x00','Byte7','0x00'),'BoardType','DS1','BoardNo',3,'ControllerNo',2),'OFF',[]}},'TLCFileName',{{'rtican_tx_message','OFF',[]}})  RTISFcnParameters=struct('SFcnRTICANMessage','struct','TLCFileName','char')  RTIBlockParaDefault=struct('BoardTypeNo',4302,'BoardNo',1,'ChannelNo',1,'Parameters',struct('DataFileSupport',struct('DataFileSelectedMaster',0,'DataFileSelectedLocal',0,'DataFileName','','DataFileDate','','SelectedFile',['<no file selected>']),'Options',struct('StatusSelected',1,'TimeSelected',1,'DeltaTimeSelected',1,'DelayTimeSelected',1,'DelayTimeTXCommandSelected',0,'EncodeSetUnusedBitsToOne',0,'EnableMsgLoopback',0,'TriggerPort',struct('Selected',0,'TriggerType','rising'),'EnablePortSelected',0,'SignalOnPortnameSelected',1,'UserCoding',struct('Selected',0,'InterfaceFile','UserEncodingFile','FcnName','UserEncodeFcn','InportSelected',0,'InportWidth',1,'OutportSelected',0,'OutportWidth',1),'TerminationMsg',struct('Selected',0,'Byte0_7','0'),'InitialMsg',struct('Selected',0,'Byte0_7','0')),'Message',struct('MsgOnBlocknameSelected',0,'MsgName',['TX Message'],'MsgIdFormat',0,'MsgId',100,'MsgLength',8,'NumSignals',1,'SampleTime',-1,'StartTime',struct('Selected',0,'Value',0),'AutoRepeatTime',struct('Selected',0,'Value',0.1),'Timeout',struct('Selected',0,'Value',0.1),'DelayTime',struct('Selected',0,'Value',0.1),'Signal',struct('SgnName',['TX signal'],'SgnStartBit',0,'SgnLength',8,'SgnType',0,'ModeValue',-1,'DataType',0,'SLDataType','SS_DOUBLE','ByteLayout',0,'Factor',1,'Offset',0,'Min',0,'Max',255,'SgnComment',{{}},'SgnUnit',''),'MsgIdNumFormat',0,'MsgComment',{{''}}),'Version',1.2,'general',struct('isFromLib',1)),'GroupId',struct('Group',{{'RTICAN'}},'No',1,'Behavior',{{'NAMECHANGE'}},'BlockType',{{'SINK'}},'NameChangeFlag',0),'SFcnRTICANMessage',struct('MsgType','TX','MsgName',['TX Message'],'MsgIdFormat','STD','MsgId',100,'MsgLength',2,'NumSignals',1,'SampleTime',-1,'StartTime',struct('Selected','no','Value',0),'AutoRepeatTime',struct('Selected','no','Value',0.1),'Timeout',struct('Selected','no','Value',0.1),'DelayTime',struct('Selected','no','Value',0.1),'Signal',struct('SgnName',['TX signal'],'SgnStartBit',0,'SgnLength',8,'SgnType','standard','ModeValue',-1,'DataType',['unsigned int'],'ByteLayout',['little endian'],'SLDataType','SS_DOUBLE','Factor',1,'Offset',0),'StatusSelected','yes','TimeSelected','yes','DeltaTimeSelected','yes','DelayTimeSelected','yes','EnablePortSelected','no','EnableMsgLoopback','no','DelayTimeTXCommandSelected','no','EncodeSetUnusedBitsToOne','no','UserCoding',struct('Selected','no','InterfaceFile','UserDecodingFile','FcnName','UserDecodeFcn','InportSelected','no','InportWidth',1,'OutportSelected','no','OutportWidth',1),'TerminationMsg',struct('Selected','no','Byte0','0x00','Byte1','0x00','Byte2','0x00','Byte3','0x00','Byte4','0x00','Byte5','0x00','Byte6','0x00','Byte7','0x00'),'InitialMsg',struct('Selected','no','Byte0','0x00','Byte1','0x00','Byte2','0x00','Byte3','0x00','Byte4','0x00','Byte5','0x00','Byte6','0x00','Byte7','0x00'),'TriggerPort',struct('Selected','no','TriggerType','rising'),'BoardType','DS4302','BoardNo',1,'ControllerNo',1,'SFcnPortType','Scalar'),'TLCFileName','rtican_tx_message')
      settings: AttributesFormatString=Group Id: RTICAN3\n  SourceProductName=dSPACE RTI CAN Blockset
  RollingCounter1 : Subsystem
  S-Function Builder1 : S-Function  InitFcn=try, set_param(gcb,'FunctionName','CheckSum_Tx_Radar410'), end  FunctionName=CheckSum_Tx_Radar410  SFunctionModules=CheckSum_Tx_Radar410_wrapper  SFunctionDeploymentMode=off  EnableBusSupport=off  mask(S-Function Builder){}
      mask help: Simulink:masks:SFunctionBuilder_MD
      mask init: same as Intergration_ACC/Tx_410_10ms/S-Function Builder1
      settings: CopyFcn=set_param(gcbh,'LinkStatus','none')  PreSaveFcn=try, set_param(gcb,'FunctionName','CheckSum_Tx_Radar410'), end  OpenFcn=sfunctionwizard(gcbh)
      mask Display: plot(val(:,1),val(:,2)),disp(sys), port_label('input',1,'data'), port_label('input',2,'length'), port_label('output',1,'u8_crc8')
  Subsystem : Subsystem
  Subsystem1 : Subsystem
  Subsystem4 : Subsystem
  Vector Concatenate1 : Concatenate  NumInputs=7
  wires:
  Constant6/1 -> S-Function Builder1/2
  Constant/1 -> Vector Concatenate1/6, Vector Concatenate1/5, Vector Concatenate1/4, Vector Concatenate1/1
  Subsystem4/1(Byte6) -> Vector Concatenate1/7
  Constant1/1 -> ESC_Status/14, ESC_Status/13, ESC_Status/12, ESC_Status/11, ESC_Status/10, ESC_Status/8, ESC_Status/7, ESC_Status/6, ESC_Status/5, ESC_Status/3, ESC_Status/4
  RollingCounter1/1(RC) -> Cast To Double2/1, Subsystem4/1(In1)
  Cast To Double2/1 -> ESC_Status/2
  Subsystem/3(Output) -> Subsystem1/1(In1)
  Subsystem1/1(Byte2) -> Vector Concatenate1/3
  <VehSpdAvg>/1 -> Subsystem/1(<WhlGndVelLDrvn_Radar>)
  Subsystem/1(Out1) -> Cast To Double4/1
  Cast To Double1/1 -> ESC_Status/1
  Vector Concatenate1/1 -> S-Function Builder1/1
  Cast To Double4/1 -> ESC_Status/9
  Subsystem/2(Byte1) -> Vector Concatenate1/2
  S-Function Builder1/1 -> Cast To Double1/1

== system Intergration_ACC/TX/RADAR_HSC2_FVCM_FrP00_0x165 ==
  RC : Inport
  COM_x165_st : Inport  Port=2
  Bus Selector1 : BusSelector  OutputSignals=ACCToqReqValHSC2,ACCToqReqStsHSC2
  Cast To Double{11..13,31} (4 alike) : DataTypeConversion  OutDataTypeStr=double
  RADAR_HSC2_FVCM_FrP00 : rtican/RTICAN Transmit (TX)   Reserved1=[]  Reserved2=[]  Reserved3=[]  Reserved4=[]  SfcnMessage=[]  Msg_Struct=[]  BoardTypeNo=[]  BoardNo=[]  ChannelNo=[]  Parameters=[]  DialogFcn=[]  UnitName=[]  Revision=[]  UnitValues=[]  DSProperties=struct('RTI',struct('Version',uint32(5),'BlockType',struct('isSLSource',uint8(1),'isSLSink',uint8(1),'isHWSource',uint8(0),'isHWSink',uint8(0),'isSetup',uint8(0),'isInline',uint8(1),'isNonInline',uint8(0),'isInterrupt',uint8(0),'isChannelwise',uint8(0)),'IOBoardType','RTICAN','UnitType','MESSAGE','Identifier','TX','DialogType','MSVC','BlockSet','RTICAN','SlaveProcessor','CAN'))  RTIBlockInterface=struct('InputPortsWidth',int32([1 1 1 1]),'InputPortsActive',[1 1 1 1],'InputPortsName',{{'ACCAlvRCHSC2','ACCToqReqValPVHSC2','ACCToqReqValHSC2','ACCToqReqStsHSC2'}},'InputPortsDataType',{{'SS_DOUBLE','SS_DOUBLE','SS_DOUBLE','SS_DOUBLE'}},'OutputPortsWidth',int32([1 1 1 1]),'OutputPortsActive',[1 1 1 1],'OutputPortsName',{{['TX status'],['TX time'],['TX delta time'],['TX delay time']}},'DialogFcn','rtican_message_interface_gui','BlockDisplay',{{'','center'}},'IconTransparency','on','InitLevel',3,'BlockName',struct('Token',{{'RADAR_HSC2_FVCM_FrP00'}}),'SampleTime',{{-1}},'TriggerPort',{{'none'}},'EnablePort',{{'none'}})  RTIBlockParameters=struct('BoardTypeNo',{{1,'OFF',[]}},'BoardNo',{{1,'ON',[1 16]}},'ChannelNo',{{1,'ON',[1 2]}},'Parameters',{{struct('DataFileSupport',struct('DataFileSelectedMaster',1,'DataFileSelectedLocal',1,'DataFileName','c:\users\administrator.zx-201607042142\desktop\zone\2020_demo\ep21原车dbc\171114-lh1-ep21_ep2_fdr-_v07.dbc|','DataFileDate',['24-11月-2020 15:06:17'],'SelectedFile','..\..\dbc\ep21_dbc\171114-lh1-ep21_ep2_fdr-_v07_acc.dbc','InterfaceFcn','rtican_dbc_file_parser'),'Options',struct('StatusSelected',1,'TimeSelected',1,'DeltaTimeSelected',1,'DelayTimeSelected',1,'DelayTimeTXCommandSelected',0,'EncodeSetUnusedBitsToOne',0,'EnableMsgLoopback',0,'TriggerPort',struct('Selected',0,'TriggerType',0),'EnablePortSelected',0,'SignalOnPortnameSelected',1,'UserCoding',struct('Selected',0,'InterfaceFile','UserEncodingFile','FcnName','UserEncodeFcn','InportSelected',0,'InportWidth',1,'OutportSelected',0,'OutportWidth',1),'TerminationMsg',struct('Selected',0,'Byte0_7','0'),'InitialMsg',struct('Selected',0,'Byte0_7','0')),'Message',struct('MsgOnBlocknameSelected',1,'MsgName','RADAR_HSC2_FVCM_FrP00','MsgIdFormat',0,'MsgId',357,'MsgLength',8,'NumSignals',4,'SampleTime',-1,'StartTime',struct('Selected',0,'Value',3),'AutoRepeatTime',struct('Selected',0,'Value',0.1),'Timeout',struct('Selected',0,'Value',0.1),'DelayTime',struct('Selected',0,'Value',0.1),'Signal',struct('SgnName',{'ACCAlvRCHSC2','ACCToqReqValPVHSC2','ACCToqReqValHSC2','ACCToqReqStsHSC2'},'SgnStartBit',{8,16,32,62},'SgnLength',{4,16,12,2},'ByteLayout',{2,2,2,2},'Factor',{1,1,2^-1,1},'Offset',{0,0,-848,0},'SgnComment',{['2017.05.23 updated:' char(10) 'ACCAEBAlvRC name changed to ACCAlvRC'],['2017.05.23 updated:' char(10) 'ACCAEBToqReqValPV name changed to ACCToqReqValPV'],['2017.05.23 updated:' char(10) 'ACCAEBToqReqVal name changed to ACCToqReqVal'],['2017.05.23 updated' char(10) 'ACCAEBToqReqSts name changed to ACCToqReqSts']},'SgnUnit',{'','','Nm',''},'Min',{0,0,-848,0},'Max',{15,65535,1199.5,3},'SgnType',{0,0,0,0},'SLDataType',{'SS_DOUBLE','SS_DOUBLE','SS_DOUBLE','SS_DOUBLE'},'DataType',{0,0,0,0},'ModeValue',{-1,-1,-1,-1}),'MsgIdNumFormat',0,'MsgComment',{{''}}),'Version',1.2,'general',struct('isFromLib',0)),'OFF',[]}},'GroupId',{{struct('Group',{{'RTICAN'}},'No',1,'Behavior',{{'NAMECHANGE'}},'BlockType',{{'SINK'}},'NameChangeFlag',0),'OFF',[]}},'SFcnRTICANMessage',{{struct('MsgType','TX','SFcnPortType','Scalar','MsgName','RADAR_HSC2_FVCM_FrP00','MsgIdFormat','STD','MsgId',357,'MsgLength',8,'NumSignals',4,'SampleTime',-1,'StartTime',struct('Selected','no','Value',3),'AutoRepeatTime',struct('Selected','no','Value',0.1),'Timeout',struct('Selected','no','Value',0.1),'Signal',struct('SgnName',{'ACCAlvRCHSC2','ACCToqReqValPVHSC2','ACCToqReqValHSC2','ACCToqReqStsHSC2'},'SgnStartBit',{8,16,32,62},'SgnLength',{4,16,12,2},'ByteLayout',{['motorola back.'],['motorola back.'],['motorola back.'],['motorola back.']},'Factor',{1,1,2^-1,1},'Offset',{0,0,-848,0},'SgnType',{'standard','standard','standard','standard'},'SLDataType',{'SS_DOUBLE','SS_DOUBLE','SS_DOUBLE','SS_DOUBLE'},'DataType',{['unsigned int'],['unsigned int'],['unsigned int'],['unsigned int']},'ModeValue',{-1,-1,-1,-1}),'StatusSelected','yes','TimeSelected','yes','DeltaTimeSelected','yes','DelayTimeSelected','yes','DelayTimeTXCommandSelected','no','EncodeSetUnusedBitsToOne','no','EnableMsgLoopback','no','TriggerPort',struct('Selected','no','TriggerType',0),'EnablePortSelected','no','UserCoding',struct('Selected','no','InterfaceFile','UserEncodingFile','FcnName','UserEncodeFcn','InportSelected','no','InportWidth',1,'OutportSelected','no','OutportWidth',1),'TerminationMsg',struct('Selected','no','Byte0','0x00','Byte1','0x00','Byte2','0x00','Byte3','0x00','Byte4','0x00','Byte5','0x00','Byte6','0x00','Byte7','0x00'),'InitialMsg',struct('Selected','no','Byte0','0x00','Byte1','0x00','Byte2','0x00','Byte3','0x00','Byte4','0x00','Byte5','0x00','Byte6','0x00','Byte7','0x00'),'BoardType','DS1','BoardNo',1,'ControllerNo',1),'OFF',[]}},'TLCFileName',{{'rtican_tx_message','OFF',[]}})  RTISFcnParameters=struct('SFcnRTICANMessage','struct','TLCFileName','char')  RTIBlockParaDefault=struct('BoardTypeNo',4302,'BoardNo',1,'ChannelNo',1,'Parameters',struct('DataFileSupport',struct('DataFileSelectedMaster',0,'DataFileSelectedLocal',0,'DataFileName','','DataFileDate','','SelectedFile',['<no file selected>']),'Options',struct('StatusSelected',1,'TimeSelected',1,'DeltaTimeSelected',1,'DelayTimeSelected',1,'DelayTimeTXCommandSelected',0,'EncodeSetUnusedBitsToOne',0,'EnableMsgLoopback',0,'TriggerPort',struct('Selected',0,'TriggerType','rising'),'EnablePortSelected',0,'SignalOnPortnameSelected',1,'UserCoding',struct('Selected',0,'InterfaceFile','UserEncodingFile','FcnName','UserEncodeFcn','InportSelected',0,'InportWidth',1,'OutportSelected',0,'OutportWidth',1),'TerminationMsg',struct('Selected',0,'Byte0_7','0'),'InitialMsg',struct('Selected',0,'Byte0_7','0')),'Message',struct('MsgOnBlocknameSelected',0,'MsgName',['TX Message'],'MsgIdFormat',0,'MsgId',100,'MsgLength',8,'NumSignals',1,'SampleTime',-1,'StartTime',struct('Selected',0,'Value',0),'AutoRepeatTime',struct('Selected',0,'Value',0.1),'Timeout',struct('Selected',0,'Value',0.1),'DelayTime',struct('Selected',0,'Value',0.1),'Signal',struct('SgnName',['TX signal'],'SgnStartBit',0,'SgnLength',8,'SgnType',0,'ModeValue',-1,'DataType',0,'SLDataType','SS_DOUBLE','ByteLayout',0,'Factor',1,'Offset',0,'Min',0,'Max',255,'SgnComment',{{}},'SgnUnit',''),'MsgIdNumFormat',0,'MsgComment',{{''}}),'Version',1.2,'general',struct('isFromLib',1)),'GroupId',struct('Group',{{'RTICAN'}},'No',1,'Behavior',{{'NAMECHANGE'}},'BlockType',{{'SINK'}},'NameChangeFlag',0),'SFcnRTICANMessage',struct('MsgType','TX','MsgName',['TX Message'],'MsgIdFormat','STD','MsgId',100,'MsgLength',2,'NumSignals',1,'SampleTime',-1,'StartTime',struct('Selected','no','Value',0),'AutoRepeatTime',struct('Selected','no','Value',0.1),'Timeout',struct('Selected','no','Value',0.1),'DelayTime',struct('Selected','no','Value',0.1),'Signal',struct('SgnName',['TX signal'],'SgnStartBit',0,'SgnLength',8,'SgnType','standard','ModeValue',-1,'DataType',['unsigned int'],'ByteLayout',['little endian'],'SLDataType','SS_DOUBLE','Factor',1,'Offset',0),'StatusSelected','yes','TimeSelected','yes','DeltaTimeSelected','yes','DelayTimeSelected','yes','EnablePortSelected','no','EnableMsgLoopback','no','DelayTimeTXCommandSelected','no','EncodeSetUnusedBitsToOne','no','UserCoding',struct('Selected','no','InterfaceFile','UserDecodingFile','FcnName','UserDecodeFcn','InportSelected','no','InportWidth',1,'OutportSelected','no','OutportWidth',1),'TerminationMsg',struct('Selected','no','Byte0','0x00','Byte1','0x00','Byte2','0x00','Byte3','0x00','Byte4','0x00','Byte5','0x00','Byte6','0x00','Byte7','0x00'),'InitialMsg',struct('Selected','no','Byte0','0x00','Byte1','0x00','Byte2','0x00','Byte3','0x00','Byte4','0x00','Byte5','0x00','Byte6','0x00','Byte7','0x00'),'TriggerPort',struct('Selected','no','TriggerType','rising'),'BoardType','DS4302','BoardNo',1,'ControllerNo',1,'SFcnPortType','Scalar'),'TLCFileName','rtican_tx_message')
      settings: AttributesFormatString=Group Id: RTICAN1\n  SourceProductName=dSPACE RTI CAN Blockset
  Subsystem4 : Subsystem
  wires:
  Bus Selector1/2 -> Subsystem4/3(ACCToqReqSts), Cast To Double12/1  "<ACCToqReqStsHSC2>"
  Cast To Double12/1 -> RADAR_HSC2_FVCM_FrP00/4
  Cast To Double31/1 -> RADAR_HSC2_FVCM_FrP00/2
  Subsystem4/2(ToqReqVal) -> Cast To Double11/1
  Bus Selector1/1 -> Subsystem4/2(ACCToqReqVal)  "<ACCToqReqValHSC2>"
  Cast To Double11/1 -> RADAR_HSC2_FVCM_FrP00/3
  Subsystem4/1(ACCToqReqValPV) -> Cast To Double31/1
  Cast To Double13/1 -> RADAR_HSC2_FVCM_FrP00/1
  COM_x165_st/1 -> Bus Selector1/1
  RC/1 -> Subsystem4/1(ACCAlvRC), Cast To Double13/1
